simulink model "link_layer_simulator"  (Simulink 7.7)
settings: Solver=ode45  StartTime=0.0  StopTime=5000.0  RelTol=1e-3
values from neighbouring files (symbols this model uses):
  use_dbpsk = dbpsk    [full_ber_curve.m]    (also in main.m = 0)
  use_rayleigh = ray    [full_ber_curve.m]    (also in main.m = 0)
libraries: commdigbbndpm3 x4, commchan3 x2, commcnvcod2 x2, commblkintrlv2 x2, commrandsrc2 x1, commsink2 x1
settings Model: Creator=skyf  LastModifiedBy=skyf

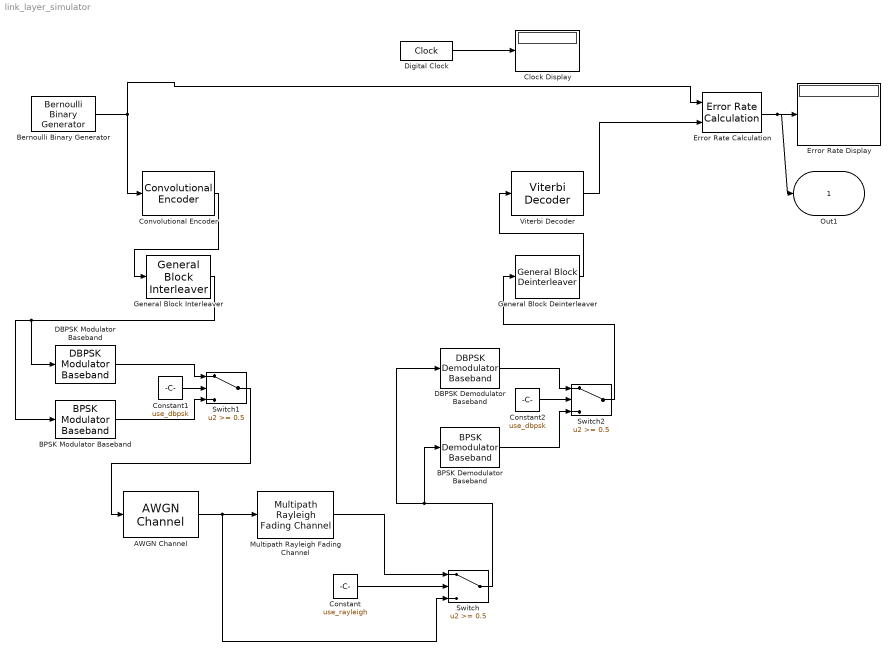
== system link_layer_simulator ==
  AWGN Channel : commchan3/AWGN Channel  SystemSampleTime=-1  InputProcessing=Columns as channels (frame based)  seed=67  noiseMode="Signal to noise ratio  (Eb/No)"  EbNodB=ebno  EsNodB=10  SNRdB=10  bitsPerSym=m  Ps=1  Tsym=1  variance=1
  BPSK Demodulator Baseband : commdigbbndpm3/BPSK Demodulator Baseband  Ph=0  DecType=Hard decision  VarSource=Dialog  Variance=1  outDtype=Inherit via internal rule  derotateFactorWordLen=16
  BPSK Modulator Baseband : commdigbbndpm3/BPSK Modulator Baseband  SystemSampleTime=-1  Ph=0  outDtype=double  outWordLen=16  outUDDataType=sfix(16)  outFracLenMode=Best precision  outFracLen=15
  Bernoulli Binary Generator : commrandsrc2/Bernoulli Binary Generator  SystemSampleTime=-1  P=0.5  seed=61  Ts=.01  frameBased=on  sampPerFrame=1000  orient=off  outDataType=boolean
  Clock Display : Display
  Constant : Constant  Value=use_rayleigh
  Constant1 : Constant  Value=use_dbpsk
  Constant2 : Constant  Value=use_dbpsk
  Convolutional Encoder : commcnvcod2/Convolutional Encoder  trellis=trellis  opMode=Truncated (reset every frame)  DelayedResetAction=off  hasIniStPort=off  hasFinStPort=off  usePuncVector=off  punctureVector=[1; 1; 0; 1; 0; 1]  reset=Unused parameter value
  DBPSK Demodulator Baseband : commdigbbndpm3/DBPSK Demodulator Baseband  SystemSampleTime=-1  Ph=0  outDtype=Inherit via internal rule
  DBPSK Modulator Baseband : commdigbbndpm3/DBPSK Modulator Baseband  SystemSampleTime=-1  Ph=0  outDtype=double
  Digital Clock : DigitalClock
  Error Rate Calculation : commsink2/Error Rate Calculation  N=0  st_delay=0  cp_mode=Entire frame  subframe=[]  PMode=Port  WsName=ErrorVec  RsMode2=off  stop=off  numErr=100  maxBits=1e6
  Error Rate Display : Display
  General Block Deinterleaver : commblkintrlv2/General Block Deinterleaver  elements=[2000:-1:1].'
  General Block Interleaver : commblkintrlv2/General Block Interleaver  elements=[2000:-1:1].'
  Multipath Rayleigh Fading Channel : commchan3/Multipath Rayleigh Fading Channel  SystemSampleTime=-1  maxDopplerShift=1  spectrumType=Jakes  sigmaGaussian=1/sqrt(2)  coeffRounded=[1 -1.72 0.785]  freqMinMaxRJakes=[0 1]  freqMinMaxAJakes=[0 1]  sigmaGaussian1=1/sqrt(2)  sigmaGaussian2=1/sqrt(2)  centerFreqGaussian1=0.0  centerFreqGaussian2=0.0  gainGaussian1=0.5  gainGaussian2=0.5  coeffBell=9  dopplerSpectrum=doppler.jakes  pathDelays=[0 2e-6]  avgPathGaindB=[0 -3]  normalizePathGains=on  seed=73  enableProbe=0  openVisAtStart=off  outPathGains=off  outDelay=off
  Switch : Switch  Threshold=0.5
  Switch1 : Switch  Threshold=0.5
  Switch2 : Switch  Threshold=0.5
  Viterbi Decoder : commcnvcod2/Viterbi Decoder  trellis=trellis  isPunctured=off  punctureVector=[1; 1; 0; 1; 0; 1]  erasures=off  dectype=Hard decision  runSigValErrCheck=off  nsdecb=2  smWordLength=16  tbdepth=39  opmode=Truncated  reset=off  outDataType=boolean
  Out1 : Outport
  wires:
  Bernoulli Binary Generator/1 -> Error Rate Calculation/1, Convolutional Encoder/1
  Error Rate Calculation/1 -> Error Rate Display/1, Out1/1
  Viterbi Decoder/1 -> Error Rate Calculation/2
  General Block Deinterleaver/1 -> Viterbi Decoder/1
  AWGN Channel/1 -> Switch/3, Multipath Rayleigh Fading Channel/1
  Constant/1 -> Switch/2
  Multipath Rayleigh Fading Channel/1 -> Switch/1
  Digital Clock/1 -> Clock Display/1
  Constant1/1 -> Switch1/2
  Convolutional Encoder/1 -> General Block Interleaver/1
  DBPSK Modulator Baseband/1 -> Switch1/1
  BPSK Modulator Baseband/1 -> Switch1/3
  Switch1/1 -> AWGN Channel/1
  General Block Interleaver/1 -> DBPSK Modulator Baseband/1, BPSK Modulator Baseband/1
  Constant2/1 -> Switch2/2
  DBPSK Demodulator Baseband/1 -> Switch2/1
  BPSK Demodulator Baseband/1 -> Switch2/3
  Switch2/1 -> General Block Deinterleaver/1
  Switch/1 -> DBPSK Demodulator Baseband/1, BPSK Demodulator Baseband/1
